simulink model "ECE414FinalProject"  (R2021a)
settings: Solver=VariableStepAuto  StartTime=0.0  StopTime=20.0  RelTol=1e-3
libraries: simulink x1
settings Model: Creator=Emily  LastModifiedBy=Emily

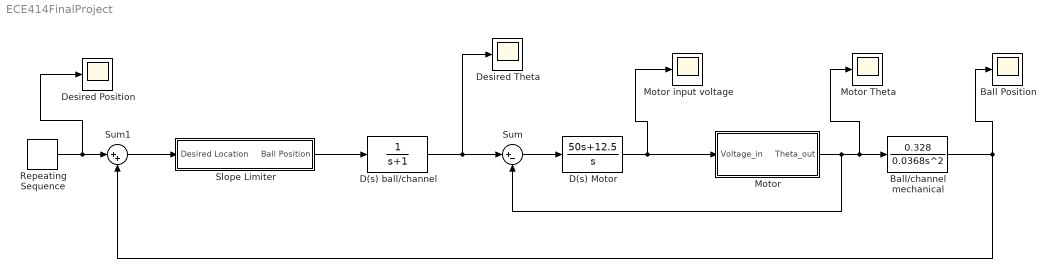
== system ECE414FinalProject ==
  Ball Position : Scope
  Ball/channel mechanical : TransferFcn  Numerator=[0.328]  Denominator=[0.0368 0 0]
  D(s) Motor : TransferFcn  Numerator=[50 12.5]  Denominator=[1 0]
  D(s) ball/channel : TransferFcn  Denominator=[1 1]
  Desired Position : Scope
  Desired Theta : Scope
  Motor : Subsystem
  Motor Theta : Scope
  Motor input voltage : Scope
  Repeating Sequence : simulink/Sources/Repeating Sequence  rep_seq_t="[0 5    5.1 10    10.1 20]"  rep_seq_y="[0 0     15 15     -20 -20]"
  Slope Limiter : Subsystem
  Sum : Sum  Inputs=|+-
  Sum1 : Sum  Inputs=|++
  wires:
  D(s) Motor/1 -> Motor input voltage/1, Motor/1(Voltage_in)
  Sum/1 -> D(s) Motor/1
  Motor/1(Theta_out) -> Motor Theta/1, Ball/channel mechanical/1, Sum/2
  Sum1/1 -> Slope Limiter/1(Desired Location)
  Ball/channel mechanical/1 -> Ball Position/1, Sum1/2
  Repeating Sequence/1 -> Desired Position/1, Sum1/1
  Slope Limiter/1(Ball Position) -> D(s) ball/channel/1
  D(s) ball/channel/1 -> Desired Theta/1, Sum/1

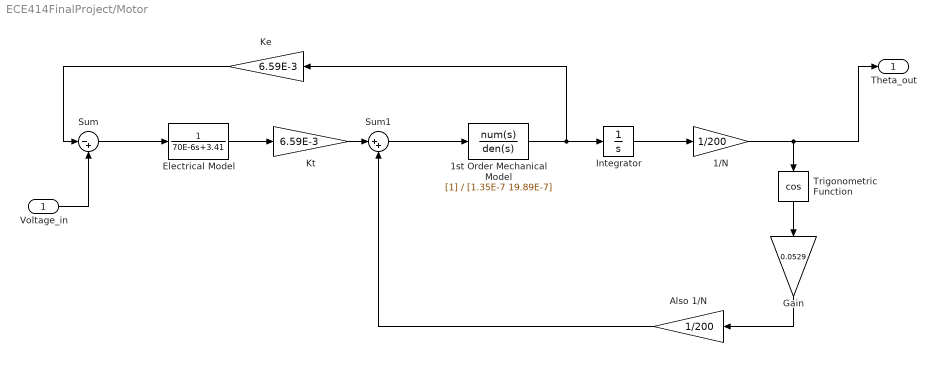
== system ECE414FinalProject/Motor ==
  Voltage_in : Inport
  1/N : Gain  Gain=1/200
  1st Order Mechanical Model : TransferFcn  Denominator=[1.35E-7 19.89E-7]
  Also 1/N : Gain  Gain=1/200
  Electrical Model : TransferFcn  Denominator=[70E-6 3.41]
  Gain : Gain  Gain=0.0529
  Integrator : Integrator
  Ke : Gain  Gain=6.59E-3
  Kt : Gain  Gain=6.59E-3
  Sum : Sum  Inputs=|-+
  Sum1 : Sum  Inputs=|++
  Trigonometric Function : Trigonometry  Operator=cos
  Theta_out : Outport
  wires:
  Ke/1 -> Sum/1
  1/N/1 -> Trigonometric Function/1, Theta_out/1
  Electrical Model/1 -> Kt/1
  1st Order Mechanical Model/1 -> Ke/1, Integrator/1
  Integrator/1 -> 1/N/1
  Also 1/N/1 -> Sum1/2
  Sum1/1 -> 1st Order Mechanical Model/1
  Kt/1 -> Sum1/1
  Sum/1 -> Electrical Model/1
  Trigonometric Function/1 -> Gain/1
  Gain/1 -> Also 1/N/1
  Voltage_in/1 -> Sum/2

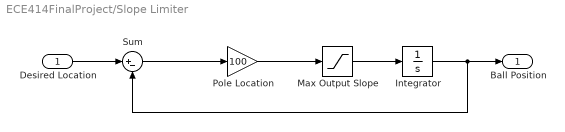
== system ECE414FinalProject/Slope Limiter ==
  Desired Location : Inport
  Integrator : Integrator
  Max Output Slope : Saturate  UpperLimit=10  LowerLimit=-10
  Pole Location : Gain  Gain=100
  Sum : Sum  Inputs=|+-
  Ball Position : Outport
  wires:
  Max Output Slope/1 -> Integrator/1
  Desired Location/1 -> Sum/1
  Sum/1 -> Pole Location/1
  Integrator/1 -> Sum/2, Ball Position/1
  Pole Location/1 -> Max Output Slope/1
